simulink model "DAB_Converter"  (R2021a)
settings: Solver=VariableStepAuto  StartTime=0.0  StopTime=10.0  RelTol=1e-3
libraries: spsIGBTDiodeLib x8, spsSeriesRLCBranchLib x2, spsDCVoltageSourceLib x1, spsLinearTransformerLib x1
settings Model: Creator=asus  LastModifiedBy=asus

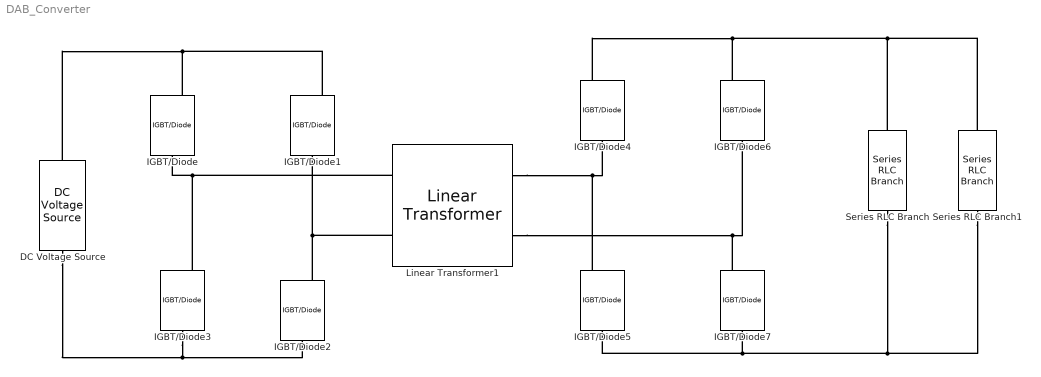
== system DAB_Converter ==
  DC Voltage Source : spsDCVoltageSourceLib/DC Voltage Source  Amplitude=100  Measurements=None
  IGBT/Diode{,1..7} (8 alike) : spsIGBTDiodeLib/IGBT//Diode  Ron=1e-3  Rs=1e5  Cs=inf  Measurements=off
  Linear Transformer1 : spsLinearTransformerLib/Linear Transformer  UNITS=SI  NominalPower=[ 50 100000 ]  winding1=[48 0 0]  winding2=[5 0 0]  ThreeWindings=off  winding3=[3.15e+05 0.7938 0.084225]  RmLm=[1.0804e+06 6.12e-3]  Measurements=None  DataType=on
  Series RLC Branch : spsSeriesRLCBranchLib/Series RLC Branch  LConnTagsString=__new0  RConnTagsString=__new0  BranchType=RC  Resistance=1  Inductance=1e-3  SetiL0=off  InitialCurrent=0  Capacitance=1e-6  Setx0=off  InitialVoltage=0  Measurements=None
  Series RLC Branch1 : spsSeriesRLCBranchLib/Series RLC Branch  LConnTagsString=__new0  RConnTagsString=__new0  BranchType=R  Resistance=1  Inductance=1e-3  SetiL0=off  InitialCurrent=0  Capacitance=1e-6  Setx0=off  InitialVoltage=0  Measurements=None
  connections:
  Linear Transformer1/LConn2 -- IGBT/Diode2/LConn1 -- IGBT/Diode1/RConn1
  Linear Transformer1/LConn1 -- IGBT/Diode/RConn1 -- IGBT/Diode3/LConn1
  DC Voltage Source/RConn1 -- IGBT/Diode1/LConn1 -- IGBT/Diode/LConn1
  DC Voltage Source/LConn1 -- IGBT/Diode3/RConn1 -- IGBT/Diode2/RConn1
  Linear Transformer1/RConn2 -- IGBT/Diode7/LConn1 -- IGBT/Diode6/RConn1
  Linear Transformer1/RConn1 -- IGBT/Diode5/LConn1 -- IGBT/Diode4/RConn1
  Series RLC Branch/RConn1 -- IGBT/Diode5/RConn1 -- IGBT/Diode7/RConn1 -- Series RLC Branch1/RConn1
  Series RLC Branch/LConn1 -- IGBT/Diode6/LConn1 -- IGBT/Diode4/LConn1 -- Series RLC Branch1/LConn1
